simulink model "stage3_rigidbody_checks"  (R2026a)
settings: Solver=ode4  FixedStep=stage3_dt
undefined symbols (not defined in the file or in its folder): stage3_contact_c, stage3_contact_force, stage3_contact_k, stage3_g, stage3_hover_thrust, stage3_Jyy, stage3_mass, stage3_normal_kd, stage3_normal_kp, stage3_probe_z, stage3_target_c, stage3_target_k, stage3_target_m
settings Model: Creator=jimmy  LastModifiedBy=jimmy

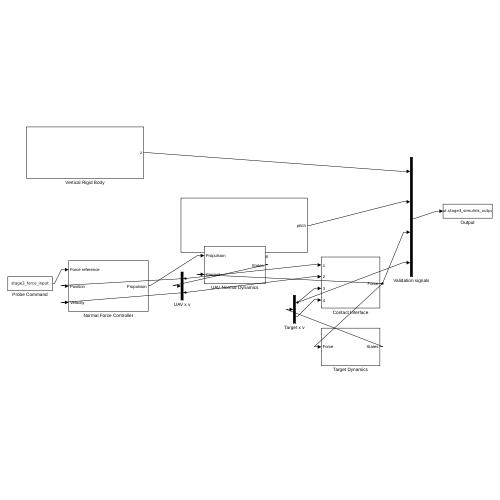
[thumbnail: Simulink's stored preview of the top-level diagram]
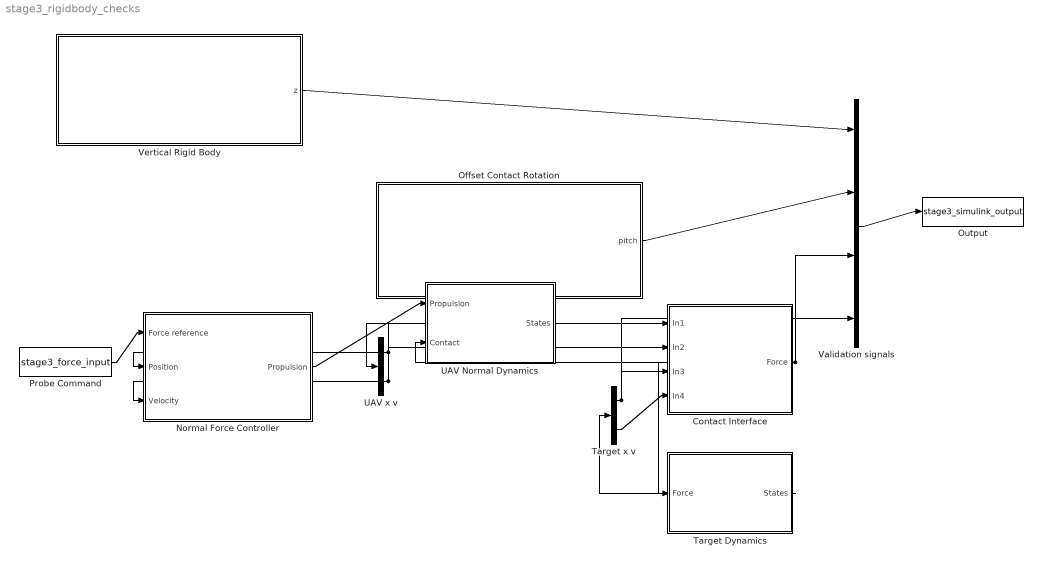
== system stage3_rigidbody_checks ==
  Contact Interface : Subsystem
  Normal Force Controller : Subsystem
  Offset Contact Rotation : Subsystem
  Output : ToWorkspace  VariableName=stage3_simulink_output  SaveFormat=Timeseries  SampleTime=-1
  Probe Command : FromWorkspace  VariableName=stage3_force_input
  Target Dynamics : Subsystem
  Target x v : Demux  Outputs=2
  UAV Normal Dynamics : Subsystem
  UAV x v : Demux  Outputs=2
  Validation signals : Mux
  Vertical Rigid Body : Subsystem
  wires:
  Probe Command/1 -> Normal Force Controller/1(Force reference)
  Normal Force Controller/1(Propulsion) -> UAV Normal Dynamics/1(Propulsion)
  Contact Interface/1(Force) -> UAV Normal Dynamics/2(Contact), Target Dynamics/1(Force), Validation signals/3
  UAV Normal Dynamics/1(States) -> UAV x v/1
  UAV x v/1 -> Normal Force Controller/2(Position), Contact Interface/1(In1)
  UAV x v/2 -> Normal Force Controller/3(Velocity), Contact Interface/2(In2)
  Target Dynamics/1(States) -> Target x v/1
  Target x v/1 -> Contact Interface/3(In3), Validation signals/4
  Target x v/2 -> Contact Interface/4(In4)
  Vertical Rigid Body/1(z) -> Validation signals/1
  Offset Contact Rotation/1(pitch) -> Validation signals/2
  Validation signals/1 -> Output/1

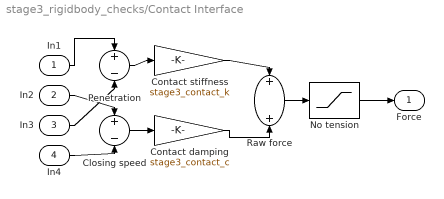
== system stage3_rigidbody_checks/Contact Interface ==
  In1 : Inport
  In2 : Inport  Port=2
  In3 : Inport  Port=3
  In4 : Inport  Port=4
  Closing speed : Sum  Inputs=+-
  Contact damping : Gain  Gain=stage3_contact_c
  Contact stiffness : Gain  Gain=stage3_contact_k
  No tension : Saturate  UpperLimit=inf  LowerLimit=0
  Penetration : Sum  Inputs=+-
  Raw force : Sum
  Force : Outport
  wires:
  In1/1 -> Penetration/1
  In3/1 -> Penetration/2
  In2/1 -> Closing speed/1
  In4/1 -> Closing speed/2
  Penetration/1 -> Contact stiffness/1
  Closing speed/1 -> Contact damping/1
  Contact stiffness/1 -> Raw force/1
  Contact damping/1 -> Raw force/2
  Raw force/1 -> No tension/1
  No tension/1 -> Force/1

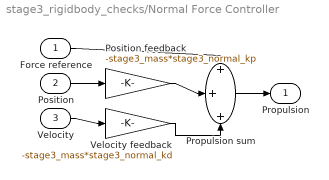
== system stage3_rigidbody_checks/Normal Force Controller ==
  Force reference : Inport
  Position : Inport  Port=2
  Velocity : Inport  Port=3
  Position feedback : Gain  Gain=-stage3_mass*stage3_normal_kp
  Propulsion sum : Sum  Inputs=+++
  Velocity feedback : Gain  Gain=-stage3_mass*stage3_normal_kd
  Propulsion : Outport
  wires:
  Force reference/1 -> Propulsion sum/1
  Position/1 -> Position feedback/1
  Velocity/1 -> Velocity feedback/1
  Position feedback/1 -> Propulsion sum/2
  Velocity feedback/1 -> Propulsion sum/3
  Propulsion sum/1 -> Propulsion/1

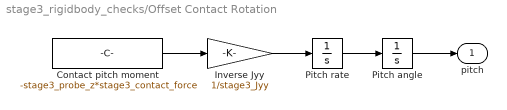
== system stage3_rigidbody_checks/Offset Contact Rotation ==
  Contact pitch moment : Constant  Value=-stage3_probe_z*stage3_contact_force
  Inverse Jyy : Gain  Gain=1/stage3_Jyy
  Pitch angle : Integrator
  Pitch rate : Integrator
  pitch : Outport
  wires:
  Contact pitch moment/1 -> Inverse Jyy/1
  Inverse Jyy/1 -> Pitch rate/1
  Pitch rate/1 -> Pitch angle/1
  Pitch angle/1 -> pitch/1

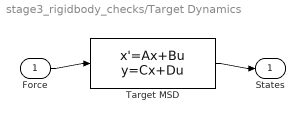
== system stage3_rigidbody_checks/Target Dynamics ==
  Force : Inport
  Target MSD : StateSpace  A=[0 1;-stage3_target_k/stage3_target_m -stage3_target_c/stage3_target_m]  B=[0;1/stage3_target_m]  C=eye(2)  D=[0;0]  InitialCondition=[0;0]
  States : Outport
  wires:
  Force/1 -> Target MSD/1
  Target MSD/1 -> States/1

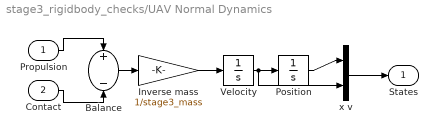
== system stage3_rigidbody_checks/UAV Normal Dynamics ==
  Propulsion : Inport
  Contact : Inport  Port=2
  Balance : Sum  Inputs=+-
  Inverse mass : Gain  Gain=1/stage3_mass
  Position : Integrator
  Velocity : Integrator
  x v : Mux  Inputs=2
  States : Outport
  wires:
  Propulsion/1 -> Balance/1
  Contact/1 -> Balance/2
  Balance/1 -> Inverse mass/1
  Inverse mass/1 -> Velocity/1
  Velocity/1 -> Position/1, x v/2
  Position/1 -> x v/1
  x v/1 -> States/1

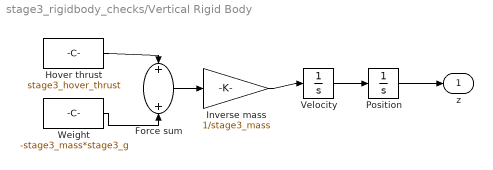
== system stage3_rigidbody_checks/Vertical Rigid Body ==
  Force sum : Sum
  Hover thrust : Constant  Value=stage3_hover_thrust
  Inverse mass : Gain  Gain=1/stage3_mass
  Position : Integrator
  Velocity : Integrator
  Weight : Constant  Value=-stage3_mass*stage3_g
  z : Outport
  wires:
  Hover thrust/1 -> Force sum/1
  Weight/1 -> Force sum/2
  Force sum/1 -> Inverse mass/1
  Inverse mass/1 -> Velocity/1
  Velocity/1 -> Position/1
  Position/1 -> z/1
